simulink model "Rober"  (Simulink 10.0)
settings: Solver=ode45  StartTime=0.0  StopTime=10.0  RelTol=1e-3  EnableMultiTasking=on
settings Model: Creator=tjohnson  LastModifiedBy=unknown
settings DataIOCC: LimitDataPoints=on
settings DebuggingCC: UnderspecifiedInitializationDetection=Simplified  MergeDetectMultiDrivingBlocksExec=error
settings GRTTargetCC: GeneratePreprocessorConditionals=Disable all  CombineOutputUpdateFcns=on  GRTInterface=off
settings ConfigComp: CovExternalEMLEnable=off

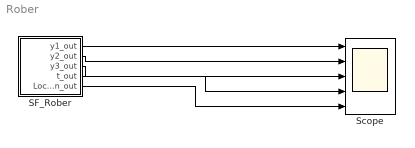
== system Rober ==
  SF_Rober : Stateflow chart  TreatAsAtomicUnit=on
  Scope : Scope  NumInputPorts=5
  wires:
  SF_Rober/1(y1_out) -> Scope/1
  SF_Rober/2(y2_out) -> Scope/2
  SF_Rober/3(y3_out) -> Scope/3
  SF_Rober/4(t_out) -> Scope/4
  SF_Rober/5(Location_out) -> Scope/5

== stateflow chart SF_Rober ==
  settings: updateMethod=CONTINUOUS
  state Rober
    du:
    y1_dot = -k1 * y1 + k3 * y2 * y3;
    y2_dot = k1 * y1 - k2 * y2 * y2 - k3 * y2 * y3;
    y3_dot = k2 * y2 ^ 2.0;
    t_dot = 1.0;
    y1_out=y1;
    y2_out=y2;
    y3_out=y3;
    t_out=t;
    Location_out =1;
  (default) -> Rober : {t = 0.0; y1 = 1.0; y2 = 0.0; y3 = 0.0;}
  data: k1 constant double =0.04; k2 constant double =30000000; k3 constant double =10000; stop_time constant double =40; y1 local double; y1_out output double; y2 local double; y2_out output double; y3 local double; y3_out output double; t local double; t_out output double; Location_out output double
  data y1 settings: updateMethod=SF_CONTINUOUS_TIME_DATA
  data y2 settings: updateMethod=SF_CONTINUOUS_TIME_DATA
  data y3 settings: updateMethod=SF_CONTINUOUS_TIME_DATA
  data t settings: updateMethod=SF_CONTINUOUS_TIME_DATA
